simulink model "PMSM"  (R2021a)
settings: Solver=ode4  StartTime=0.0  StopTime=4  FixedStep=1e-5  RelTol=1e-3
values from neighbouring files (symbols this model uses):
  Ki = We*rs    (= 12.5663706144)    [Param1.m]
  Kp = We*Lq    (= 0.0188495559215)    [Param1.m]
  Lambda_m_r = 0.01    [Param1.m]
  Ld = 300e-6    (= 0.0003)    [Param1.m]    (also in Param2.m = 0.00016)
  Ll = 0.01*272e-6    (= 2.72e-06)    [Param1.m]
  Lm = (2/3) * Lq    (= 0.0002)    [Param1.m]
  Lq = 300e-6    (= 0.0003)    [Param1.m]    (also in Param2.m = 0.00016)
  rs = 0.2    [Param1.m]
libraries: spsControlledVoltageSourceLib x6, spsCurrentMeasurementLib x3, spsGroundLib x1, spsMutualInductanceLib x1, spspowerguiLib x1
settings Model: Creator=clinic  LastModifiedBy=clinic

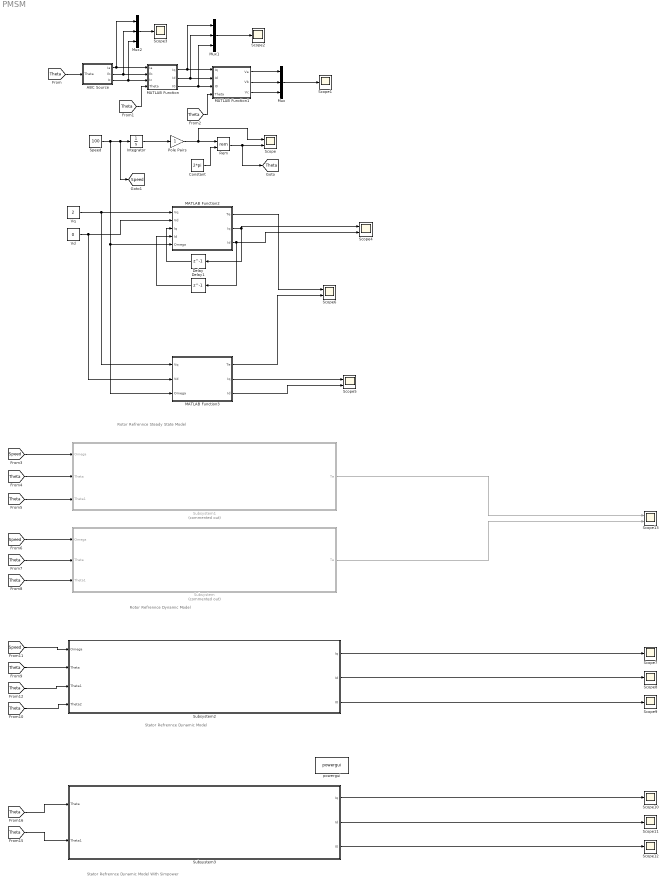
== system PMSM ==
  note: Rotor Refrennce Dynamic Model
  note: Rotor Refrennce Steady State Model
  note: Stator Refrennce Dynamic Model
  note: Stator Refrennce Dynamic Model With Simpower
  ABC Source : MATLAB Function  TreatAsAtomicUnit=on
  Constant : Constant  Value=2*pi
  Delay : Delay  DelayLength=1
  Delay1 : Delay  DelayLength=1
  Integrator : Integrator
  MATLAB Function : MATLAB Function  TreatAsAtomicUnit=on
  MATLAB Function1 : MATLAB Function  TreatAsAtomicUnit=on
  MATLAB Function2 : MATLAB Function  TreatAsAtomicUnit=on
  MATLAB Function3 : MATLAB Function  TreatAsAtomicUnit=on
  Mux : Mux  Inputs=3
  Mux1 : Mux  Inputs=3
  Mux2 : Mux  Inputs=3
  Pole Pairs : Gain
  Rem : Math  Operator=rem  SaturateOnIntegerOverflow=on
  Scope{,4..6,13} (5 alike) : Scope  NumInputPorts=2
  Scope{1..3,7..12} (9 alike) : Scope
  Speed : Constant  Value=100
  Subsystem : Subsystem  Commented=on
  Subsystem1 : Subsystem  Commented=on
  Subsystem2 : Subsystem
  Subsystem3 : Subsystem
  Vd : Constant  Value=0
  Vq : Constant  Value=2
  powergui : spspowerguiLib/powergui  Priority=1  SimulationMode=Continuous  SampleTime=50e-6  frequency=60  Iterations=50  frequencyindice=0  Pbase=100e6  ErrMax=1e-4  UnitsV=kV  UnitsW=MW  buscounter=0  FunctionMessages=off  echomessages=off  EnableUseOfTLC=off  CurrentSourceSwitches=off  DisableSnubberDevices=off  DisableRonSwitches=off  DisableVfSwitches=off  DisplayEquations=off  AutomaticDiscreteSolvers=off  SolverType=Tustin/Backward Euler (TBE)  Interpol=off  ExternalGateDelay=off  methode=off  Ts=100  x0status=blocks  SPID=on  SwTol=0  HookPort=off  NonlinearTolerance=1e-4  nMaxIteration=100  ContinueOnMaxIteration=off  RestoreLinks=warning  ResistiveCurrentMeasurement=off  Frange=[0:2:500]  Ylog=off  Xlog=on  ShowGrid=off  save=off  variable=ZData  structure=0  ZoomFFT=off  StartTime=0.0  cycles=1  DisplayStyle=1  fundamental=60  FreqAxis=off  MaxFrequency=1000  frequencyindicesteady=1  RmsSteady=1  display=off
  tag scope: Speed=global, Theta=global
  wires:
  Integrator/1 -> Pole Pairs/1
  Pole Pairs/1 -> Scope/1, Rem/1
  Constant/1 -> Rem/2
  Rem/1 -> [Theta], Scope/2
  [Theta] -> ABC Source/1(Theta)
  ABC Source/1(Ia) -> Mux2/1, MATLAB Function/1(Ia)
  ABC Source/2(Ib) -> Mux2/2, MATLAB Function/2(Ib)
  ABC Source/3(Ic) -> MATLAB Function/3(Ic), Mux2/3
  [Theta] -> MATLAB Function/4(Theta)
  MATLAB Function/1(Iq) -> Mux1/1, MATLAB Function1/1(Iq)
  MATLAB Function/2(Id) -> Mux1/2, MATLAB Function1/2(Id)
  MATLAB Function/3(I0) -> Mux1/3, MATLAB Function1/3(I0)
  [Theta] -> MATLAB Function1/4(Theta)
  MATLAB Function1/1(Va) -> Mux/1
  MATLAB Function1/2(Vb) -> Mux/2
  MATLAB Function1/3(Vc) -> Mux/3
  Mux/1 -> Scope1/1
  Mux1/1 -> Scope2/1
  Mux2/1 -> Scope3/1
  Vq/1 -> MATLAB Function3/1(Vq), MATLAB Function2/1(Vq)
  Vd/1 -> MATLAB Function3/2(Vd), MATLAB Function2/2(Vd)
  MATLAB Function2/2(Iq) -> Scope4/1, Delay/1
  Delay/1 -> MATLAB Function2/3("Iq ")
  MATLAB Function2/3(Id) -> Delay1/1, Scope4/2
  Delay1/1 -> MATLAB Function2/4("Id ")
  Speed/1 -> MATLAB Function3/3(Omega), MATLAB Function2/5(Omega), [Speed], Integrator/1
  MATLAB Function3/2(Iq) -> Scope5/1
  MATLAB Function3/3(Id) -> Scope5/2
  MATLAB Function2/1(Te) -> Scope6/1
  MATLAB Function3/1(Te) -> Scope6/2
  [Speed] -> Subsystem/1(Omega)
  [Theta] -> Subsystem/2(Theta)
  [Theta] -> Subsystem/3(Theta1)
  Subsystem/1(Te) -> Scope13/2
  [Speed] -> Subsystem1/1(Omega)
  [Theta] -> Subsystem1/2(Theta)
  [Theta] -> Subsystem1/3(Theta1)
  Subsystem1/1(Te) -> Scope13/1
  [Speed] -> Subsystem2/1(Omega)
  [Theta] -> Subsystem2/2(Theta)
  [Theta] -> Subsystem2/3(Theta1)
  [Theta] -> Subsystem2/4(Theta2)
  Subsystem2/1(Iq) -> Scope7/1
  Subsystem2/2(Id) -> Scope8/1
  Subsystem2/3(I0) -> Scope9/1
  [Theta] -> Subsystem3/2(Theta1)
  Subsystem3/1(Iq) -> Scope10/1
  [Theta] -> Subsystem3/1(Theta)
  Subsystem3/3(I0) -> Scope12/1
  Subsystem3/2(Id) -> Scope11/1

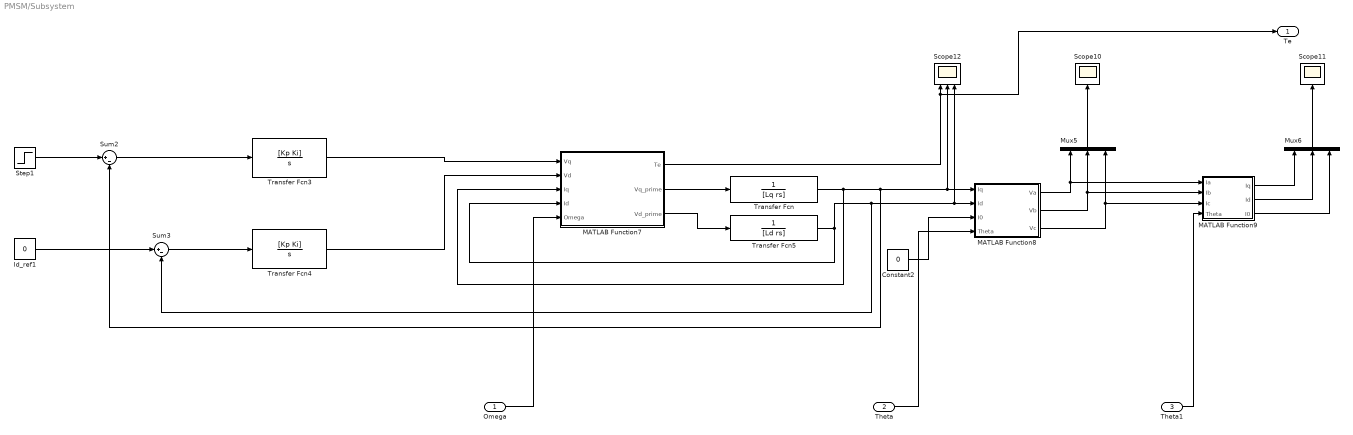
== system PMSM/Subsystem ==
  Omega : Inport
  Theta : Inport  Port=2
  Theta1 : Inport  Port=3
  Constant2 : Constant  Value=0
  Id_ref1 : Constant  Value=0
  MATLAB Function7 : MATLAB Function  TreatAsAtomicUnit=on
  MATLAB Function8 : MATLAB Function  TreatAsAtomicUnit=on
  MATLAB Function9 : MATLAB Function  TreatAsAtomicUnit=on
  Mux5 : Mux  Inputs=3
  Mux6 : Mux  Inputs=3
  Scope10 : Scope
  Scope11 : Scope
  Scope12 : Scope  NumInputPorts=3
  Step1 : Step  Time=2  After=2  SampleTime=0
  Sum2 : Sum  Inputs=|+-
  Sum3 : Sum  Inputs=|+-
  Transfer Fcn : TransferFcn  Denominator=[Lq rs]
  Transfer Fcn3 : TransferFcn  Numerator=[Kp Ki]  Denominator=[1 0]
  Transfer Fcn4 : TransferFcn  Numerator=[Kp Ki]  Denominator=[1 0]
  Transfer Fcn5 : TransferFcn  Denominator=[Ld rs]
  Te : Outport
  wires:
  Transfer Fcn/1 -> MATLAB Function7/3(Iq), MATLAB Function8/1(Iq), Scope12/2, Sum2/2
  Transfer Fcn3/1 -> MATLAB Function7/1(Vq)
  MATLAB Function8/2(Vb) -> MATLAB Function9/2(Ib), Mux5/2
  MATLAB Function7/2(Vq_prime) -> Transfer Fcn/1
  MATLAB Function9/3(I0) -> Mux6/3
  Transfer Fcn5/1 -> MATLAB Function7/4(Id), Sum3/2, Scope12/3, MATLAB Function8/2(Id)
  Step1/1 -> Sum2/1
  MATLAB Function8/1(Va) -> MATLAB Function9/1(Ia), Mux5/1
  MATLAB Function7/3(Vd_prime) -> Transfer Fcn5/1
  Transfer Fcn4/1 -> MATLAB Function7/2(Vd)
  MATLAB Function9/1(Iq) -> Mux6/1
  Theta1/1 -> MATLAB Function9/4(Theta)
  MATLAB Function8/3(Vc) -> MATLAB Function9/3(Ic), Mux5/3
  Mux5/1 -> Scope10/1
  Omega/1 -> MATLAB Function7/5(Omega)
  MATLAB Function9/2(Id) -> Mux6/2
  Mux6/1 -> Scope11/1
  Constant2/1 -> MATLAB Function8/3(I0)
  MATLAB Function7/1(Te) -> Te/1, Scope12/1
  Sum3/1 -> Transfer Fcn4/1
  Sum2/1 -> Transfer Fcn3/1
  Id_ref1/1 -> Sum3/1
  Theta/1 -> MATLAB Function8/4(Theta)

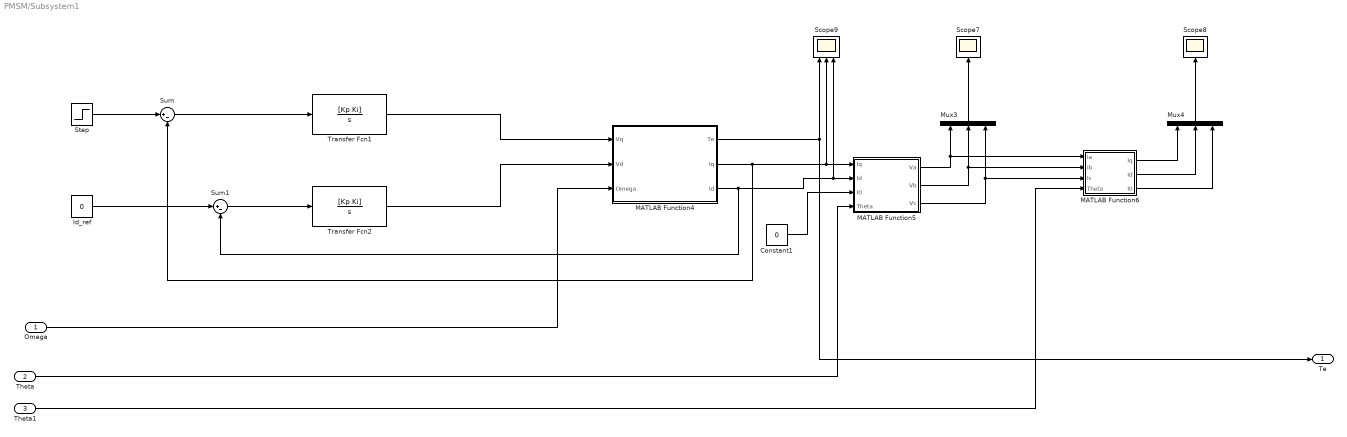
== system PMSM/Subsystem1 ==
  Omega : Inport
  Theta : Inport  Port=2
  Theta1 : Inport  Port=3
  Constant1 : Constant  Value=0
  Id_ref : Constant  Value=0
  MATLAB Function4 : MATLAB Function  TreatAsAtomicUnit=on
  MATLAB Function5 : MATLAB Function  TreatAsAtomicUnit=on
  MATLAB Function6 : MATLAB Function  TreatAsAtomicUnit=on
  Mux3 : Mux  Inputs=3
  Mux4 : Mux  Inputs=3
  Scope7 : Scope
  Scope8 : Scope
  Scope9 : Scope  NumInputPorts=3
  Step : Step  Time=2  After=2  SampleTime=0
  Sum : Sum  Inputs=|+-
  Sum1 : Sum  Inputs=|+-
  Transfer Fcn1 : TransferFcn  Numerator=[Kp Ki]  Denominator=[1 0]
  Transfer Fcn2 : TransferFcn  Numerator=[Kp Ki]  Denominator=[1 0]
  Te : Outport
  wires:
  Constant1/1 -> MATLAB Function5/3(I0)
  MATLAB Function5/2(Vb) -> MATLAB Function6/2(Ib), Mux3/2
  Step/1 -> Sum/1
  MATLAB Function6/2(Id) -> Mux4/2
  MATLAB Function6/1(Iq) -> Mux4/1
  Sum/1 -> Transfer Fcn1/1
  MATLAB Function4/2(Iq) -> Sum/2, MATLAB Function5/1(Iq), Scope9/2
  MATLAB Function4/3(Id) -> Sum1/2, Scope9/3, MATLAB Function5/2(Id)
  Sum1/1 -> Transfer Fcn2/1
  Mux4/1 -> Scope8/1
  Transfer Fcn1/1 -> MATLAB Function4/1(Vq)
  Omega/1 -> MATLAB Function4/3(Omega)
  MATLAB Function6/3(I0) -> Mux4/3
  Transfer Fcn2/1 -> MATLAB Function4/2(Vd)
  Theta/1 -> MATLAB Function5/4(Theta)
  MATLAB Function5/3(Vc) -> MATLAB Function6/3(Ic), Mux3/3
  MATLAB Function4/1(Te) -> Te/1, Scope9/1
  MATLAB Function5/1(Va) -> MATLAB Function6/1(Ia), Mux3/1
  Id_ref/1 -> Sum1/1
  Theta1/1 -> MATLAB Function6/4(Theta)
  Mux3/1 -> Scope7/1

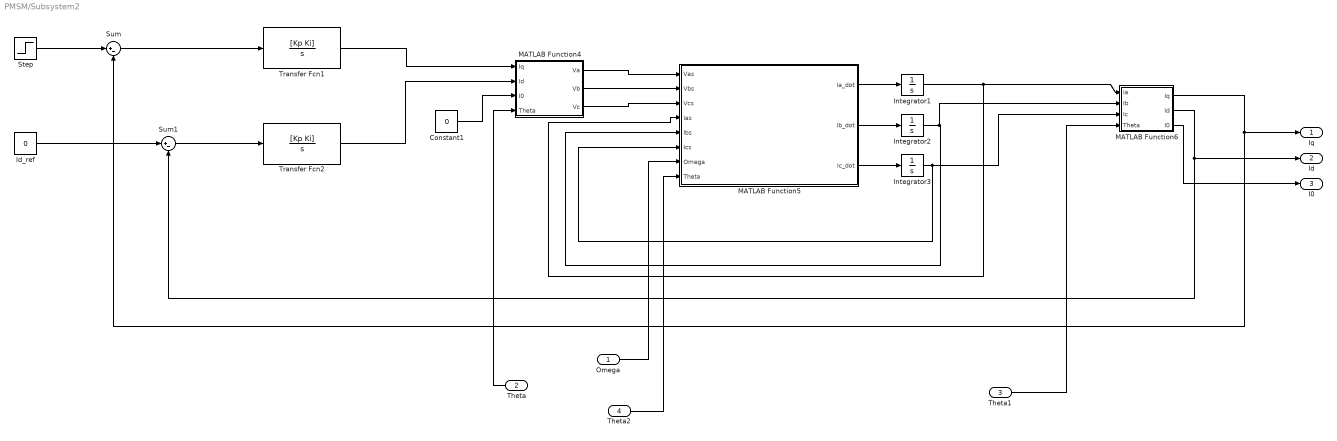
== system PMSM/Subsystem2 ==
  Omega : Inport
  Theta : Inport  Port=2
  Theta1 : Inport  Port=3
  Theta2 : Inport  Port=4
  Constant1 : Constant  Value=0
  Id_ref : Constant  Value=0
  Integrator1 : Integrator
  Integrator2 : Integrator
  Integrator3 : Integrator
  MATLAB Function4 : MATLAB Function  TreatAsAtomicUnit=on
  MATLAB Function5 : MATLAB Function  TreatAsAtomicUnit=on
  MATLAB Function6 : MATLAB Function  TreatAsAtomicUnit=on
  Step : Step  Time=2  After=2  SampleTime=0
  Sum : Sum  Inputs=|+-
  Sum1 : Sum  Inputs=|+-
  Transfer Fcn1 : TransferFcn  Numerator=[Kp Ki]  Denominator=[1 0]
  Transfer Fcn2 : TransferFcn  Numerator=[Kp Ki]  Denominator=[1 0]
  Iq : Outport
  Id : Outport  Port=2
  I0 : Outport  Port=3
  wires:
  MATLAB Function6/1(Iq) -> Iq/1, Sum/2
  Transfer Fcn2/1 -> MATLAB Function4/2(Id)
  MATLAB Function6/2(Id) -> Id/1, Sum1/2
  MATLAB Function5/3(Ic_dot) -> Integrator3/1
  Integrator3/1 -> MATLAB Function5/6(Ics), MATLAB Function6/3(Ic)
  Transfer Fcn1/1 -> MATLAB Function4/1(Iq)
  Integrator2/1 -> MATLAB Function6/2(Ib), MATLAB Function5/5(Ibs)
  MATLAB Function4/2(Vb) -> MATLAB Function5/2(Vbs)
  Theta/1 -> MATLAB Function4/4(Theta)
  MATLAB Function4/1(Va) -> MATLAB Function5/1(Vas)
  Constant1/1 -> MATLAB Function4/3(I0)
  MATLAB Function5/2(Ib_dot) -> Integrator2/1
  Integrator1/1 -> MATLAB Function5/4(Ias), MATLAB Function6/1(Ia)
  MATLAB Function5/1(Ia_dot) -> Integrator1/1
  MATLAB Function4/3(Vc) -> MATLAB Function5/3(Vcs)
  Sum1/1 -> Transfer Fcn2/1
  Step/1 -> Sum/1
  Sum/1 -> Transfer Fcn1/1
  Id_ref/1 -> Sum1/1
  MATLAB Function6/3(I0) -> I0/1
  Theta2/1 -> MATLAB Function5/8(Theta)
  Omega/1 -> MATLAB Function5/7(Omega)
  Theta1/1 -> MATLAB Function6/4(Theta)

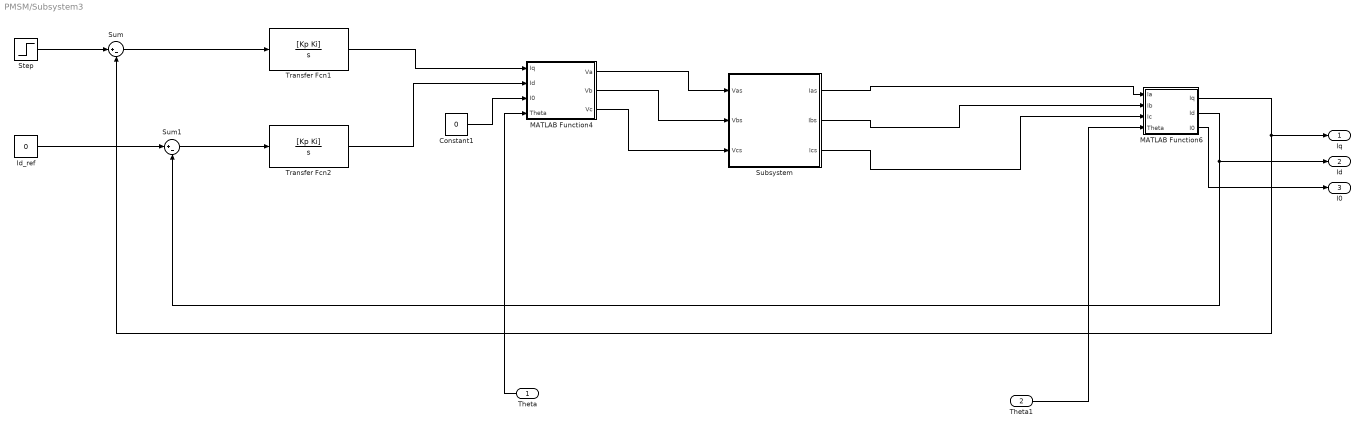
== system PMSM/Subsystem3 ==
  Theta : Inport
  Theta1 : Inport  Port=2
  Constant1 : Constant  Value=0
  Id_ref : Constant  Value=0
  MATLAB Function4 : MATLAB Function  TreatAsAtomicUnit=on
  MATLAB Function6 : MATLAB Function  TreatAsAtomicUnit=on
  Step : Step  Time=2  After=2  SampleTime=0
  Subsystem : Subsystem
  Sum : Sum  Inputs=|+-
  Sum1 : Sum  Inputs=|+-
  Transfer Fcn1 : TransferFcn  Numerator=[Kp Ki]  Denominator=[1 0]
  Transfer Fcn2 : TransferFcn  Numerator=[Kp Ki]  Denominator=[1 0]
  Iq : Outport
  Id : Outport  Port=2
  I0 : Outport  Port=3
  wires:
  MATLAB Function6/1(Iq) -> Iq/1, Sum/2
  Transfer Fcn2/1 -> MATLAB Function4/2(Id)
  MATLAB Function6/2(Id) -> Id/1, Sum1/2
  Subsystem/3(Ics) -> MATLAB Function6/3(Ic)
  Transfer Fcn1/1 -> MATLAB Function4/1(Iq)
  Subsystem/2(Ibs) -> MATLAB Function6/2(Ib)
  MATLAB Function4/2(Vb) -> Subsystem/2(Vbs)
  Theta/1 -> MATLAB Function4/4(Theta)
  MATLAB Function4/1(Va) -> Subsystem/1(Vas)
  Constant1/1 -> MATLAB Function4/3(I0)
  Subsystem/1(Ias) -> MATLAB Function6/1(Ia)
  MATLAB Function4/3(Vc) -> Subsystem/3(Vcs)
  Sum1/1 -> Transfer Fcn2/1
  Step/1 -> Sum/1
  Sum/1 -> Transfer Fcn1/1
  Id_ref/1 -> Sum1/1
  MATLAB Function6/3(I0) -> I0/1
  Theta1/1 -> MATLAB Function6/4(Theta)

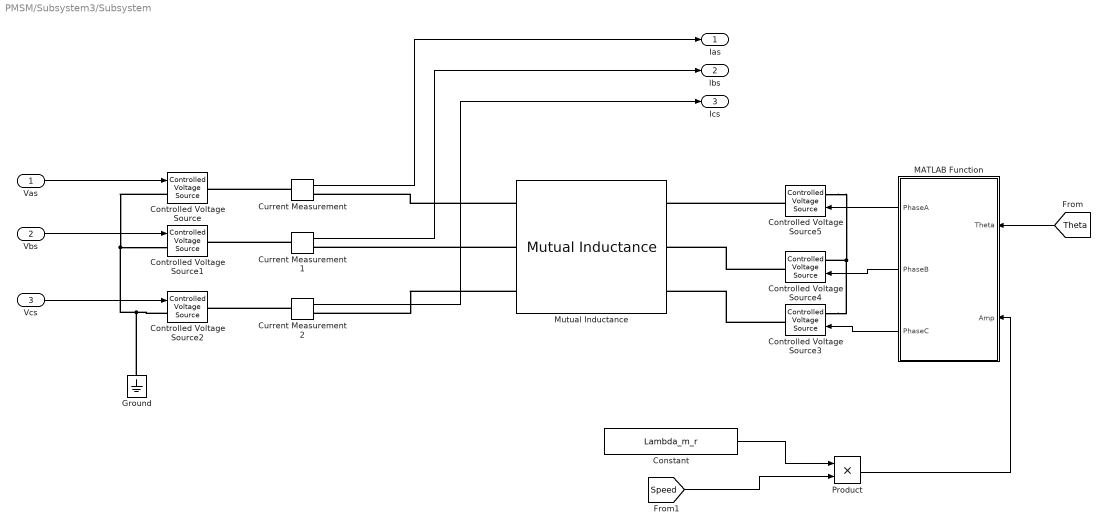
== system PMSM/Subsystem3/Subsystem ==
  Vas : Inport
  Vbs : Inport  Port=2
  Vcs : Inport  Port=3
  Constant : Constant  Value=Lambda_m_r
  Controlled Voltage Source{,1..5} (6 alike) : spsControlledVoltageSourceLib/Controlled Voltage Source  Initialize=on  Source_Type=AC  Amplitude=0  Phase=0  Frequency=0  Measurements=None
  Current Measurement : spsCurrentMeasurementLib/Current Measurement  PhasorSimulation=off  OutputType=Complex  PSBequivalent=0
  Current Measurement1 : spsCurrentMeasurementLib/Current Measurement  PhasorSimulation=off  OutputType=Complex  PSBequivalent=0
  Current Measurement2 : spsCurrentMeasurementLib/Current Measurement  PhasorSimulation=off  OutputType=Complex  PSBequivalent=0
  Ground : spsGroundLib/Ground  LConnTagsString=a
  MATLAB Function : MATLAB Function  TreatAsAtomicUnit=on
  Mutual Inductance : spsMutualInductanceLib/Mutual Inductance  LConnTagsString=a|b|c  RConnTagsString=A|B|C  TypeOfMutual=Generalized mutual inductance  NumberOfWindings=3  SelfImpedance1=[1.1 1.1e-03]  SelfImpedance2=[ 1.1 1.1e-03]  ThreeWindings=on  SelfImpedance3=[ 1.1 1.1e-03]  MutualImpedance=[1.0 1.0e-03]  InductanceMatrix=[Ll+Lm -0.5*Lm -0.5*Lm;-0.5*Lm Ll+Lm -0.5*Lm;-0.5*Lm -0.5*Lm Ll+Lm]  ResistanceMatrix="[rs 0 0;0  rs 0;0  0  rs]"  Measurements=None
      settings: SourceProductBaseCode=PS
  Product : Product
  Ias : Outport
  Ibs : Outport  Port=2
  Ics : Outport  Port=3
  wires:
  Vas/1 -> Controlled Voltage Source/1
  Vbs/1 -> Controlled Voltage Source1/1
  Vcs/1 -> Controlled Voltage Source2/1
  MATLAB Function/1(PhaseA) -> Controlled Voltage Source5/1
  MATLAB Function/2(PhaseB) -> Controlled Voltage Source4/1
  MATLAB Function/3(PhaseC) -> Controlled Voltage Source3/1
  [Theta] -> MATLAB Function/1(Theta)
  Constant/1 -> Product/1
  [Speed] -> Product/2
  Product/1 -> MATLAB Function/2(Amp)
  Current Measurement/1 -> Ias/1
  Current Measurement1/1 -> Ibs/1
  Current Measurement2/1 -> Ics/1
  connections:
  Current Measurement/LConn1 -- Controlled Voltage Source/RConn1
  Controlled Voltage Source/LConn1 -- Controlled Voltage Source1/LConn1 -- Controlled Voltage Source2/LConn1 -- Ground/LConn1
  Current Measurement1/LConn1 -- Controlled Voltage Source1/RConn1
  Current Measurement2/LConn1 -- Controlled Voltage Source2/RConn1
  Mutual Inductance/LConn1 -- Current Measurement/RConn1
  Mutual Inductance/LConn2 -- Current Measurement1/RConn1
  Mutual Inductance/LConn3 -- Current Measurement2/RConn1
  Controlled Voltage Source5/RConn1 -- Mutual Inductance/RConn1
  Controlled Voltage Source4/RConn1 -- Mutual Inductance/RConn2
  Controlled Voltage Source3/RConn1 -- Mutual Inductance/RConn3
  Controlled Voltage Source5/LConn1 -- Controlled Voltage Source3/LConn1 -- Controlled Voltage Source4/LConn1

== matlab function PMSM/Subsystem/MATLAB Function7 ==
  data: Vq input; Te output; Vd input; Iq input; Id input; Omega input; Vq_prime output; Vd_prime output
function [Te,Vq_prime,Vd_prime] = fcn(Vq,Vd,Iq,Id,Omega)
rs = 0.2;
Lq = 300e-6;
Ld = 300e-6;
Lambda_m_r = 0.01;
p = 2;

Vq_prime= Vq - Omega*Ld*Id - Omega*Lambda_m_r
Vd_prime = Vd + Omega*Lq*Iq
Te = (3/2)*(p/2)*(Lambda_m_r*Iq+(Ld-Lq)*Iq*Id);

== matlab function PMSM/Subsystem/MATLAB Function8 ==
  data: Iq input; Va output; Id input; I0 input; Theta input; Vb output; Vc output
function [Va,Vb,Vc] = fcn(Iq,Id,I0,Theta)
Va = cos(Theta)*Iq + sin(Theta)*Id +1*I0;
Vb = cos(Theta-2*pi/3)*Iq + sin(Theta-2*pi/3)*Id +1*I0;
Vc = cos(Theta+2*pi/3)*Iq + sin(Theta+2*pi/3)*Id +1*I0;

== matlab function PMSM/Subsystem/MATLAB Function9 ==
  data: Ia input; Iq output; Ib input; Ic input; Theta input; Id output; I0 output
function [Iq,Id,I0] = fcn(Ia,Ib,Ic,Theta)
Iq = 2/3*( cos(Theta)*Ia + cos(Theta-2*pi/3)*Ib + cos(Theta+2*pi/3)*Ic );
Id = 2/3*( sin(Theta)*Ia + sin(Theta-2*pi/3)*Ib + sin(Theta+2*pi/3)*Ic );
I0 = 2/3*( 1/2*Ia + 1/2*Ib + 1/2*Ic );

== matlab function PMSM/Subsystem2/MATLAB Function4 ==
  data: Iq input; Va output; Id input; I0 input; Theta input; Vb output; Vc output
function [Va,Vb,Vc] = fcn(Iq,Id,I0,Theta)
Va = cos(Theta)*Iq + sin(Theta)*Id +1*I0;
Vb = cos(Theta-2*pi/3)*Iq + sin(Theta-2*pi/3)*Id +1*I0;
Vc = cos(Theta+2*pi/3)*Iq + sin(Theta+2*pi/3)*Id +1*I0;

== matlab function PMSM/Subsystem2/MATLAB Function5 ==
  data: Vas input; Ia_dot output; Vbs input; Vcs input; Ias input; Ibs input; Ics input; Omega input; Theta input; Ib_dot output; Ic_dot output
function [Ia_dot,Ib_dot,Ic_dot] = fcn(Vas,Vbs,Vcs,Ias,Ibs,Ics,Omega,Theta)
rs = 0.2;
Lq = 300e-6;
Ld = 300e-6;
Lambda_m_r = 0.01;
p = 2;
Lm = (2/3) * Lq;
Ll = 0.01*272e-6;
Rs = [rs 0 0;
      0  rs 0;
      0  0  rs];
Vs = [Vas;Vbs;Vcs];
Ind = [Ll+Lm -0.5*Lm -0.5*Lm;
       -0.5*Lm Ll+Lm -0.5*Lm;
       -0.5*Lm -0.5*Lm Ll+Lm];

Bemf = [Lambda_m_r*Omega*cos(Theta);
        Lambda_m_r*Omega*cos(Theta-2*pi/3);
        Lambda_m_r*Omega*cos(Theta+2*pi/3)];
I= [Ias; Ibs; Ics];
Ans = (inv(Ind)) * ((Vs - Rs*I) - Bemf);
Ia_dot = Ans(1);
Ib_dot = Ans(2);
Ic_dot = Ans(3);

== matlab function PMSM/MATLAB Function ==
  data: Ia input; Iq output; Ib input; Ic input; Theta input; Id output; I0 output
function [Iq,Id,I0] = fcn(Ia,Ib,Ic,Theta)
Iq = 2/3*( cos(Theta)*Ia + cos(Theta-2*pi/3)*Ib + cos(Theta+2*pi/3)*Ic );
Id = 2/3*( sin(Theta)*Ia + sin(Theta-2*pi/3)*Ib + sin(Theta+2*pi/3)*Ic );
I0 = 2/3*( 1/2*Ia + 1/2*Ib + 1/2*Ic );

== matlab function PMSM/Subsystem2/MATLAB Function6 ==
  data: Ia input; Iq output; Ib input; Ic input; Theta input; Id output; I0 output
function [Iq,Id,I0] = fcn(Ia,Ib,Ic,Theta)
Iq = 2/3*( cos(Theta)*Ia + cos(Theta-2*pi/3)*Ib + cos(Theta+2*pi/3)*Ic );
Id = 2/3*( sin(Theta)*Ia + sin(Theta-2*pi/3)*Ib + sin(Theta+2*pi/3)*Ic );
I0 = 2/3*( 1/2*Ia + 1/2*Ib + 1/2*Ic );

== matlab function PMSM/Subsystem3/MATLAB Function4 ==
  data: Iq input; Va output; Id input; I0 input; Theta input; Vb output; Vc output
function [Va,Vb,Vc] = fcn(Iq,Id,I0,Theta)
Va = cos(Theta)*Iq + sin(Theta)*Id +1*I0;
Vb = cos(Theta-2*pi/3)*Iq + sin(Theta-2*pi/3)*Id +1*I0;
Vc = cos(Theta+2*pi/3)*Iq + sin(Theta+2*pi/3)*Id +1*I0;

== matlab function PMSM/Subsystem3/Subsystem/MATLAB Function ==
  data: Theta input; PhaseA output; Amp input; PhaseB output; PhaseC output
function [PhaseA, PhaseB, PhaseC] = fcn(Theta, Amp)
PhaseA  = Amp * cos(Theta);
PhaseB  = Amp * cos(Theta-2*pi/3);
PhaseC  = Amp * cos(Theta+2*pi/3);

== matlab function PMSM/Subsystem3/MATLAB Function6 ==
  data: Ia input; Iq output; Ib input; Ic input; Theta input; Id output; I0 output
function [Iq,Id,I0] = fcn(Ia,Ib,Ic,Theta)
Iq = 2/3*( cos(Theta)*Ia + cos(Theta-2*pi/3)*Ib + cos(Theta+2*pi/3)*Ic );
Id = 2/3*( sin(Theta)*Ia + sin(Theta-2*pi/3)*Ib + sin(Theta+2*pi/3)*Ic );
I0 = 2/3*( 1/2*Ia + 1/2*Ib + 1/2*Ic );

== matlab function PMSM/ABC Source ==
  data: Theta input; Ia output; Ib output; Ic output
function [Ia,Ib,Ic] = fcn(Theta)
Ia = sin(Theta);
Ib = sin(Theta-2*pi/3);
Ic = sin(Theta+2*pi/3);

== matlab function PMSM/MATLAB Function1 ==
  data: Iq input; Va output; Id input; I0 input; Theta input; Vb output; Vc output
function [Va,Vb,Vc] = fcn(Iq,Id,I0,Theta)
Va = cos(Theta)*Iq + sin(Theta)*Id +1*I0;
Vb = cos(Theta-2*pi/3)*Iq + sin(Theta-2*pi/3)*Id +1*I0;
Vc = cos(Theta+2*pi/3)*Iq + sin(Theta+2*pi/3)*Id +1*I0;

== matlab function PMSM/MATLAB Function2 ==
  data: Vq input; Te output; Vd input; Iq input; Id input; Omega input; Iq output; Id output
function [Te,Iq,Id] = fcn(Vq,Vd,Iq,Id,Omega)
rs = 0.2;
Lq = 300e-6;
Ld = 300e-6;
Lambda_m_r = 0.01;
p = 2;

Iq = (1/rs)*(Vq - Omega*Ld*Id - Omega*Lambda_m_r);
Id = (1/rs)*(Vd + Omega*Lq*Iq);
Te = (3/2)*(p/2)*(Lambda_m_r*Iq+(Ld-Lq)*Iq*Id);

== matlab function PMSM/MATLAB Function3 ==
  data: Vq input; Vd input; Te output; Omega input; Iq output; Id output
function [Te,Iq,Id] = fcn(Vq,Vd,Omega)
rs = 0.2;
Lq = 300e-6;
Ld = 300e-6;
Lambda_m_r = 0.01;
p = 2;

k= rs^2 + (Omega^2)*Lq*Ld;

Iq = (rs/k) * (Vq-Omega*Lambda_m_r-Omega*Ld*Vd/rs);
Id = (rs/k) * (Vd+Omega*Lq*Vq/rs-(Omega^2)*Lq*Lambda_m_r/rs)
Te = (3/2)*(p/2)*(Lambda_m_r*Iq+(Ld-Lq)*Iq*Id);

== matlab function PMSM/Subsystem1/MATLAB Function4 ==
  data: Vq input; Vd input; Te output; Omega input; Iq output; Id output
function [Te,Iq,Id] = fcn(Vq,Vd,Omega)
rs = 0.2;
Lq = 300e-6;
Ld = 300e-6;
Lambda_m_r = 0.01;
p = 2;

k= rs^2 + (Omega^2)*Lq*Ld;

Iq = (rs/k) * (Vq-Omega*Lambda_m_r-Omega*Ld*Vd/rs);
Id = (rs/k) * (Vd+Omega*Lq*Vq/rs-(Omega^2)*Lq*Lambda_m_r/rs)
Te = (3/2)*(p/2)*(Lambda_m_r*Iq+(Ld-Lq)*Iq*Id);

== matlab function PMSM/Subsystem1/MATLAB Function5 ==
  data: Iq input; Va output; Id input; I0 input; Theta input; Vb output; Vc output
function [Va,Vb,Vc] = fcn(Iq,Id,I0,Theta)
Va = cos(Theta)*Iq + sin(Theta)*Id +1*I0;
Vb = cos(Theta-2*pi/3)*Iq + sin(Theta-2*pi/3)*Id +1*I0;
Vc = cos(Theta+2*pi/3)*Iq + sin(Theta+2*pi/3)*Id +1*I0;

== matlab function PMSM/Subsystem1/MATLAB Function6 ==
  data: Ia input; Iq output; Ib input; Ic input; Theta input; Id output; I0 output
function [Iq,Id,I0] = fcn(Ia,Ib,Ic,Theta)
Iq = 2/3*( cos(Theta)*Ia + cos(Theta-2*pi/3)*Ib + cos(Theta+2*pi/3)*Ic );
Id = 2/3*( sin(Theta)*Ia + sin(Theta-2*pi/3)*Ib + sin(Theta+2*pi/3)*Ic );
I0 = 2/3*( 1/2*Ia + 1/2*Ib + 1/2*Ic );
